simulink model "main"  (R2025b)
settings: Solver=ode1  StartTime=0.0  StopTime=config.sim.var.sim_time  FixedStep=config.sim.var.time_step  RelTol=1e-3
PreLoadFcn:
  | addpath(fullfile(pwd,'images'));
InitFcn:
  | run(fullfile(fileparts(get_param(bdroot,'FileName')),'initializer.mlx'))
StopFcn:
  | run(fullfile(fileparts(get_param(bdroot,'FileName')),'plot/plotting_results.m'))
undefined symbols (not defined in the file): config
libraries: simulink x8, sharedTrackingLibrary x2
(part 2 of 2)

== matlab function main/Controller/Non Linear Controller - Feedback Linearisation/Virtual Controller ==
  settings: updateMethod=DISCRETE  sampleTime=config.sim.var.time_step
  data: e_i output; Ref_d input; x_est input; v output; config parameter
function [e_i, v] = fcn(Ref_d, x_est, config)

    % States desired position
    q_d = Ref_d(1:2);
    dot_q_d = Ref_d(3:4);
    ddot_q_d = Ref_d(5:6);
    
    % States
    q = x_est(1:2);
    dot_q = x_est(3:4);
    
    % Controller Config
    action = config.sim.mode.controllerConfig.action;
    payload = config.sim.mode.controllerConfig.payloadCompensation;

    % For I controller
    % e_i error (is reseted in config_params file in initialization)
    persistent e_i_prev 

    if isempty(e_i_prev) 
        e_i_prev = zeros(2,1);
    end
    
    % time step
    dt = config.contrl.non_linear_fdbck_lin.param.I_controller.intStep; % integrator step the same as simulation step
    
    % Errors:
    e_p = q_d - q;
    e_d = dot_q_d - dot_q;
    
    if (action == ControllerAction.PID_zeta_omega) || (action == ControllerAction.PID_LQR)
        e_i = e_i_prev + e_p*dt;
    else
        e_i = e_i_prev;
    end
    
    % clamping e_i (min/max)
    e_i_max = config.contrl.non_linear_fdbck_lin.param.I_controller.clamp_max;
    e_i = min(max(e_i, -e_i_max), e_i_max);

    % Saving integral error for next integration
    e_i_prev = e_i;
 
    
    
    % Chosing gains based on: action and payload
    % Chosing gains based on: action and payload
    if (payload == ControllerPayloadCompensation.NotActive)
    
        switch action
            case ControllerAction.PD_zeta_omega
                k_p = config.contrl.non_linear_fdbck_lin.no_payload.PD_zeta_omega.gains.k_p;
                k_d = config.contrl.non_linear_fdbck_lin.no_payload.PD_zeta_omega.gains.k_d;
                k_i = diag([0;0]);
    
            case ControllerAction.PD_LQR
                k_p = config.contrl.non_linear_fdbck_lin.no_payload.PD_LQR.gains.k_p;
                k_d = config.contrl.non_linear_fdbck_lin.no_payload.PD_LQR.gains.k_d;
                k_i = diag([0;0]);
    
            case ControllerAction.PID_zeta_omega
                k_p = config.contrl.non_linear_fdbck_lin.no_payload.PID_zeta_omega.gains.k_p;
                k_d = config.contrl.non_linear_fdbck_lin.no_payload.PID_zeta_omega.gains.k_d;
                k_i = config.contrl.non_linear_fdbck_lin.no_payload.PID_zeta_omega.gains.k_i;
            case ControllerAction.PID_LQR
                k_p = config.contrl.non_linear_fdbck_lin.no_payload.PID_LQR.gains.k_p;
                k_d = config.contrl.non_linear_fdbck_lin.no_payload.PID_LQR.gains.k_d;
                k_i = config.contrl.non_linear_fdbck_lin.no_payload.PID_LQR.gains.k_i;
            otherwise
                error("Unsupported ControllerAction for no-payload mode");
        end
    
    elseif (payload == ControllerPayloadCompensation.Active)
    
        switch action
            case ControllerAction.PD_zeta_omega
                k_p = config.contrl.non_linear_fdbck_lin.payload.PD_zeta_omega.gains.k_p;
                k_d = config.contrl.non_linear_fdbck_lin.payload.PD_zeta_omega.gains.k_d;
                k_i = diag([0;0]);
    
            case ControllerAction.PD_LQR
                k_p = config.contrl.non_linear_fdbck_lin.payload.PD_LQR.gains.k_p;
                k_d = config.contrl.non_linear_fdbck_lin.payload.PD_LQR.gains.k_d;
                k_i = diag([0;0]);
    
            case ControllerAction.PID_zeta_omega
                k_p = config.contrl.non_linear_fdbck_lin.payload.PID_zeta_omega.gains.k_p;
                k_d = config.contrl.non_linear_fdbck_lin.payload.PID_zeta_omega.gains.k_d;
                k_i = config.contrl.non_linear_fdbck_lin.payload.PID_zeta_omega.gains.k_i;
            case ControllerAction.PID_LQR
                k_p = config.contrl.non_linear_fdbck_lin.payload.PID_LQR.gains.k_p;
                k_d = config.contrl.non_linear_fdbck_lin.payload.PID_LQR.gains.k_d;
                k_i = config.contrl.non_linear_fdbck_lin.payload.PID_LQR.gains.k_i;
            otherwise
                error("Unsupported ControllerAction for no-payload mode");
        end
    
    else
        error("Unsupported controllerConfig.payloadCompensation value");
    end

    
    v = ddot_q_d + k_p*e_p + k_d*e_d + k_i*e_i;
end

== matlab function main/Controller/Non Linear Controller - Feedback Linearisation/Feedback Linearisation ==
  data: v input; x_est input; u output; config parameter
function u = fcn(v, x_est, config)

% states
q = x_est(1:2);
dot_q = x_est(3:4);

% Control law
payload = config.sim.mode.controllerConfig.payloadCompensation;

if payload == ControllerPayloadCompensation.NotActive
    u = (M(q, config)*v + c_vec(q, dot_q, config) + G_vec(q, config) + D_mat(config)*dot_q);
elseif payload == ControllerPayloadCompensation.Active
    m_ext =config.contrl.non_linear_fdbck_lin.payload.mass;
    W = [0;
        -m_ext*9.81];
    u = M(q, config)*v + c_vec(q, dot_q, config) + G_vec(q, config) + D_mat(config)*dot_q - J_T(q, config)*W;
else
    error("Unsupported controllerConfig Payload combination");
end

== matlab function main/State Observability/State Reconstruction Dirty Derivative/Mux like func (for great support for exporting var) ==
  data: q1 input; x_est output; q2 input; dot_q1 input; dot_q2 input
function x_est = fcn(q1, q2, dot_q1, dot_q2)

x_est = [q1;
         q2;
         dot_q1;
         dot_q2];

== matlab function main/State Observability/State Reconstruction Derivative with Low Pass Filter/Mux like func (for great support for exporting var) ==
  data: q1 input; x_est output; q2 input; dot_q1 input; dot_q2 input
function x_est = fcn(q1, q2, dot_q1, dot_q2)

x_est = [q1;
         q2;
         dot_q1;
         dot_q2];

== matlab function main/State Observability/Extended Kalman Filter/Mux like func (for great support for exporting var) ==
  data: q1 input; x_est output; q2 input; dot_q1 input; dot_q2 input
function x_est = fcn(q1, q2, dot_q1, dot_q2)

x_est = [q1;
         q2;
         dot_q1;
         dot_q2];
